simulink model "Filter"  (R2020b)
settings: Solver=VariableStepAuto  StartTime=0.0  StopTime=10.0  RelTol=1e-3
settings Model: Creator=smart  LastModifiedBy=smart

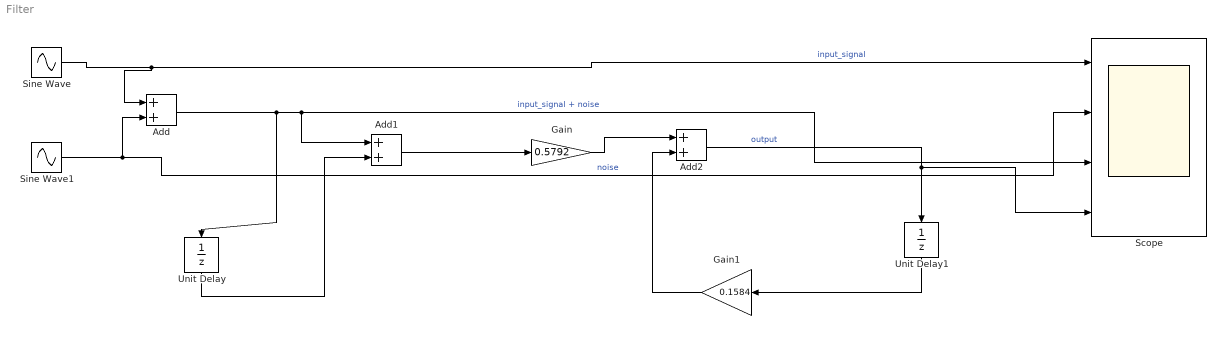
== system Filter ==
  Add : Sum
  Add1 : Sum
  Add2 : Sum
  Gain : Gain  Gain=0.5792
  Gain1 : Gain  Gain=0.1584
  Scope : Scope  NumInputPorts=4
  Sine Wave : Sin  SampleTime=0
  Sine Wave1 : Sin  Amplitude=0.5  Frequency=50  SampleTime=0
  Unit Delay : UnitDelay  SampleTime=-1  HasFrameUpgradeWarning=on
  Unit Delay1 : UnitDelay  SampleTime=-1  HasFrameUpgradeWarning=on
  wires:
  Sine Wave/1 -> Scope/1, Add/1  "input_signal"
  Sine Wave1/1 -> Scope/2, Add/2  "noise"
  Add2/1 -> Scope/4, Unit Delay1/1  "output"
  Unit Delay1/1 -> Gain1/1
  Gain1/1 -> Add2/2
  Gain/1 -> Add2/1
  Add1/1 -> Gain/1
  Add/1 -> Scope/3, Add1/1, Unit Delay/1  "input_signal + noise"
  Unit Delay/1 -> Add1/2
